simulink model "Lab1PartC4"  (R2023b)
settings: Solver=VariableStepAuto  StartTime=0.0  StopTime=3  RelTol=1e-3
settings Model: Creator=mathe  LastModifiedBy=mathe

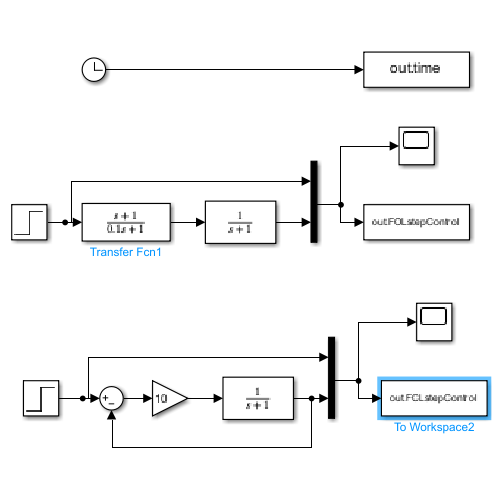
[thumbnail: Simulink's stored preview of the top-level diagram]
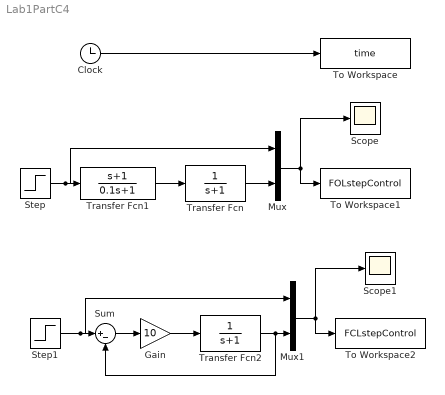
== system Lab1PartC4 ==
  Clock : Clock
      settings: Decimation=100
  Gain : Gain  Gain=10
  Mux : Mux  Inputs=2
  Mux1 : Mux  Inputs=2
  Scope : Scope
  Scope1 : Scope
  Step : Step  Time=0  SampleTime=0
  Step1 : Step  Time=0  SampleTime=0
  Sum : Sum  Inputs=|+-
  To Workspace : ToWorkspace  VariableName=time  SampleTime=-1
  To Workspace1 : ToWorkspace  VariableName=FOLstepControl  SampleTime=-1
  To Workspace2 : ToWorkspace  VariableName=FCLstepControl  SampleTime=-1
  Transfer Fcn : TransferFcn  Denominator=[1 1]
  Transfer Fcn1 : TransferFcn  Numerator=[1 1]  Denominator=[0.1 1]
  Transfer Fcn2 : TransferFcn  Denominator=[1 1]
  wires:
  Mux1/1 -> To Workspace2/1, Scope1/1
  Step1/1 -> Mux1/1, Sum/1
  Transfer Fcn2/1 -> Sum/2, Mux1/2
  Step/1 -> Mux/1, Transfer Fcn1/1
  Sum/1 -> Gain/1
  Transfer Fcn1/1 -> Transfer Fcn/1
  Gain/1 -> Transfer Fcn2/1
  Mux/1 -> To Workspace1/1, Scope/1
  Transfer Fcn/1 -> Mux/2
  Clock/1 -> To Workspace/1
